simulink model "CUQNUTTALL"  (R2024b)
settings: Solver=ode15s  StartTime=0.0  StopTime=0.2  RelTol=1e-3
values from neighbouring files (symbols this model uses):
  b = 8.5e-3    (= 0.0085)    [TD2_config.m]    (also in TD3_config.m)
  Cr = 0    [TD2_config.m]    (also in TD3_config.m)
  J = 0.28    [TD2_config.m]    (also in TD3_config.m)
  K = Km    (= 0.5093)    [TD2_config.m]    (also in TD3_config.m)
  L = 1.6e-3    (= 0.0016)    [TD2_config.m]    (also in TD3_config.m)
  R = 0.13    [TD2_config.m]    (also in TD3_config.m)
  U = 12    [TD2_config.m]    (also in TD3_config.m)
settings Model: Creator=E306_PC2  LastModifiedBy=E306_PC2

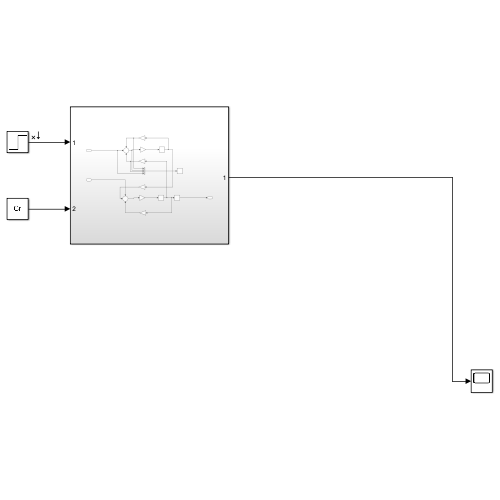
[thumbnail: Simulink's stored preview of the top-level diagram]
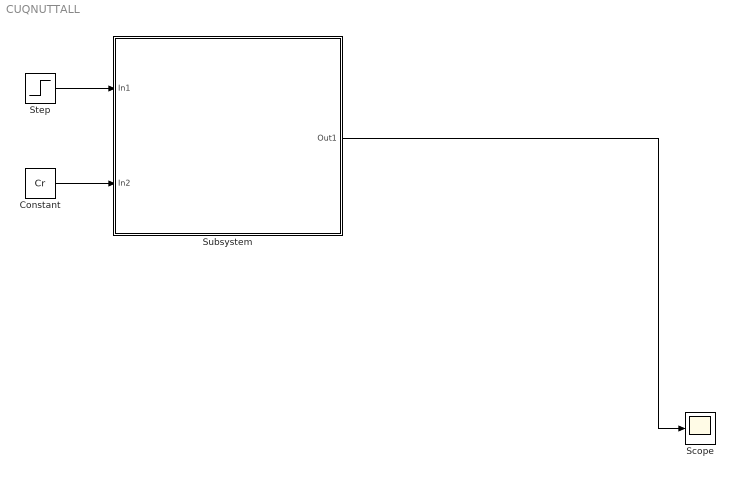
== system CUQNUTTALL ==
  Constant : Constant  Value=Cr
  Scope : Scope
  Step : Step  Time=0  After=U  SampleTime=0
  Subsystem : Subsystem
  wires:
  Step/1 -> Subsystem/1(In1)
  Constant/1 -> Subsystem/2(In2)
  Subsystem/1(Out1) -> Scope/1

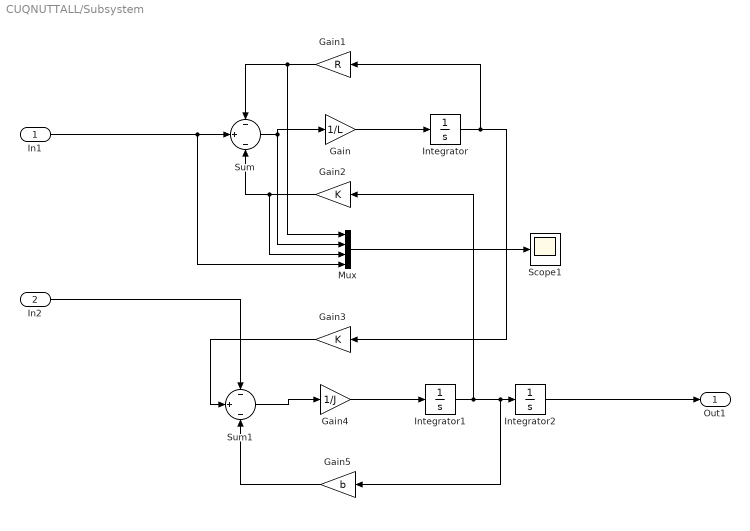
== system CUQNUTTALL/Subsystem ==
  In1 : Inport
  In2 : Inport  Port=2
  Gain : Gain  Gain=1/L
  Gain1 : Gain  Gain=R
  Gain2 : Gain  Gain=K
  Gain3 : Gain  Gain=K
  Gain4 : Gain  Gain=1/J
  Gain5 : Gain  Gain=b
  Integrator : Integrator
  Integrator1 : Integrator
  Integrator2 : Integrator
  Mux : Mux
  Scope1 : Scope
  Sum : Sum  Inputs=-|+|-
  Sum1 : Sum  Inputs=-|+|-
  Out1 : Outport
  wires:
  Integrator2/1 -> Out1/1
  Mux/1 -> Scope1/1
  Gain2/1 -> Mux/3, Sum/3
  Integrator1/1 -> Integrator2/1, Gain5/1, Gain2/1
  Gain1/1 -> Mux/1, Sum/1
  Gain5/1 -> Sum1/3
  Integrator/1 -> Gain1/1, Gain3/1
  In1/1 -> Mux/4, Sum/2
  Sum/1 -> Gain/1, Mux/2
  Gain4/1 -> Integrator1/1
  Gain/1 -> Integrator/1
  Gain3/1 -> Sum1/2
  Sum1/1 -> Gain4/1
  In2/1 -> Sum1/1
